simulink library "calc_path_coordinates"  (R2022a)
settings: Solver=VariableStepAuto  StartTime=0.0  StopTime=10.0  RelTol=1e-3
settings Model: Creator=Ayaz  LastModifiedBy=lhill8
settings SolverCC: AlgebraicLoopSolver=TrustRegion
settings DebuggingCC: UnconnectedInputMsg=warning  UnconnectedOutputMsg=warning  UnconnectedLineMsg=warning  SFMachineParentedDataDiag=warning

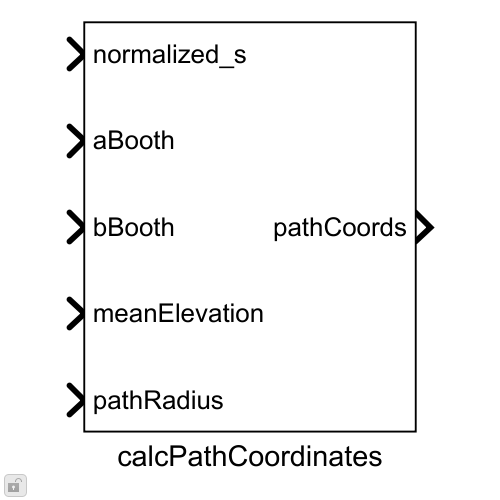
[thumbnail: Simulink's stored preview of the top-level diagram]
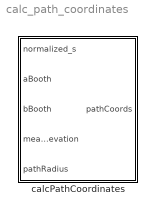
== system calc_path_coordinates ==
  calcPathCoordinates : Subsystem

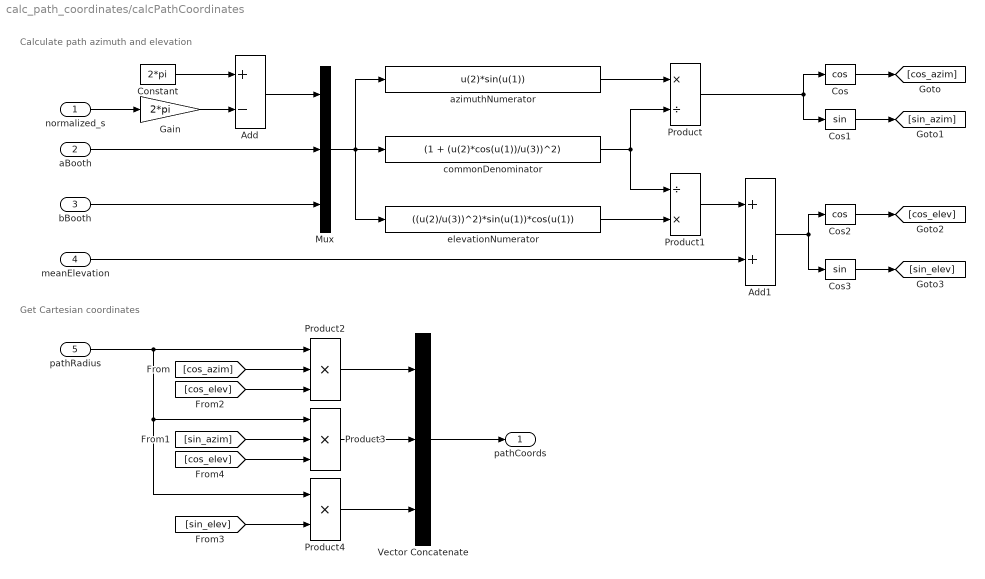
== system calc_path_coordinates/calcPathCoordinates ==
  note: Calculate path azimuth and elevation
  note: Get Cartesian coordinates
  normalized_s : Inport
  aBooth : Inport  Port=2
  bBooth : Inport  Port=3
  meanElevation : Inport  Port=4
  pathRadius : Inport  Port=5
  Add : Sum  Inputs=+-
  Add1 : Sum
  Constant : Constant  Value=2*pi
  Cos : Trigonometry  Operator=cos
  Cos1 : Trigonometry
  Cos2 : Trigonometry  Operator=cos
  Cos3 : Trigonometry
  Gain : Gain  Gain=2*pi
  Mux : Mux  Inputs=3
  Product : Product  Inputs=*/
  Product1 : Product  Inputs=/*
  Product2 : Product  Inputs=3
  Product3 : Product  Inputs=3
  Product4 : Product
  Vector Concatenate : Concatenate  NumInputs=3
  azimuthNumerator : Fcn  Expr=u(2)*sin(u(1))
  commonDenominator : Fcn  Expr=(1 + (u(2)*cos(u(1))/u(3))^2)
  elevationNumerator : Fcn  Expr=((u(2)/u(3))^2)*sin(u(1))*cos(u(1))
  pathCoords : Outport
  wires:
  Gain/1 -> Add/2
  aBooth/1 -> Mux/2
  bBooth/1 -> Mux/3
  Mux/1 -> elevationNumerator/1, azimuthNumerator/1, commonDenominator/1
  Constant/1 -> Add/1
  normalized_s/1 -> Gain/1
  Add/1 -> Mux/1
  azimuthNumerator/1 -> Product/1
  commonDenominator/1 -> Product/2, Product1/1
  elevationNumerator/1 -> Product1/2
  Product1/1 -> Add1/1
  meanElevation/1 -> Add1/2
  Product/1 -> Cos1/1, Cos/1
  Cos/1 -> [cos_azim]
  Cos1/1 -> [sin_azim]
  Cos2/1 -> [cos_elev]
  Cos3/1 -> [sin_elev]
  Add1/1 -> Cos2/1, Cos3/1
  [cos_azim] -> Product2/2
  [cos_elev] -> Product2/3
  pathRadius/1 -> Product2/1, Product4/1, Product3/1
  [sin_azim] -> Product3/2
  [cos_elev] -> Product3/3
  [sin_elev] -> Product4/2
  Product2/1 -> Vector Concatenate/1
  Product3/1 -> Vector Concatenate/2
  Product4/1 -> Vector Concatenate/3
  Vector Concatenate/1 -> pathCoords/1
